simulink model "sine_wave_detect_15"  (R2021a)
settings: Solver=FixedStepAuto  StartTime=0.0  StopTime=10.0  FixedStep=1e-3  RelTol=1e-3
settings Model: Creator=yasso  LastModifiedBy=yasso

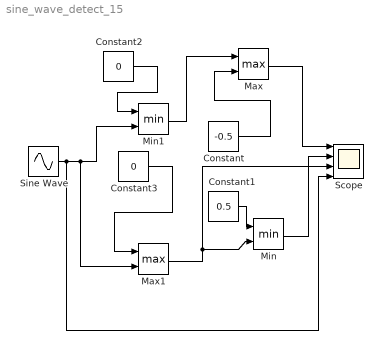
== system sine_wave_detect_15 ==
  Constant : Constant  Value=-0.5
  Constant1 : Constant  Value=0.5
  Constant2 : Constant  Value=0
  Constant3 : Constant  Value=0
  Max : MinMax  Function=max  Inputs=2
  Max1 : MinMax  Function=max  Inputs=2
  Min : MinMax  Inputs=2
  Min1 : MinMax  Inputs=2
  Scope : Scope  NumInputPorts=4
  Sine Wave : Sin  SampleTime=0
  wires:
  Sine Wave/1 -> Scope/4, Max1/2, Min1/2
  Constant/1 -> Max/2
  Min1/1 -> Max/1
  Constant1/1 -> Min/1
  Max1/1 -> Scope/3, Min/2
  Min/1 -> Scope/2
  Max/1 -> Scope/1
  Constant2/1 -> Min1/1
  Constant3/1 -> Max1/1
